simulink model "SingleWheelAug"  (R2025b)
settings: Solver=VariableStepAuto  StartTime=0.0  StopTime=10.0  RelTol=1e-3
undefined symbols (not defined in the file): InvDyn, ureal, uss
libraries: RCTblocks x2
settings Model: Creator=d.alazard  LastModifiedBy=andre
settings SolverCC: AlgebraicLoopSolver=TrustRegion
settings DebuggingCC: AlgebraicLoopMsg=none  UnconnectedInputMsg=warning  UnconnectedOutputMsg=warning  UnconnectedLineMsg=warning
settings ModelReferenceCC: EnableRefExpFcnMdlSchedulingChecks=on
settings RTWCC: GPUComputeCapability=3.5  DLArmComputeVersion=19.05

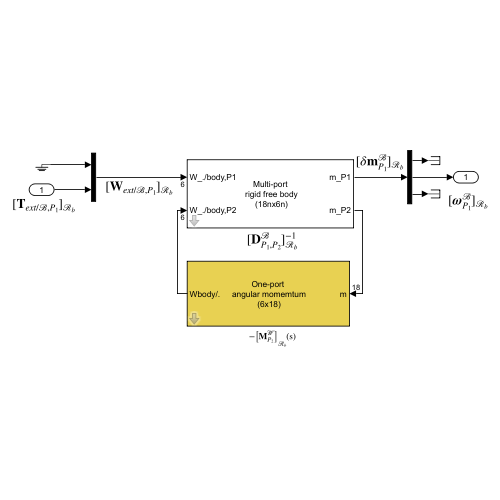
[thumbnail: Simulink's stored preview of the top-level diagram]
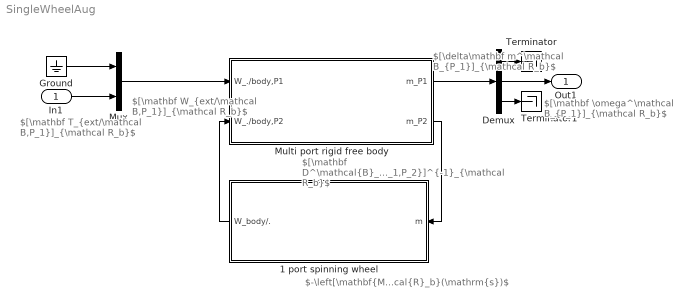
== system SingleWheelAug ==
  note: $-\left[\mathbf{M}^{\mathcal{W}}_{P_2}\right]_{\mathcal{R}_b}(\mathrm{s})$
  note: $[\mathbf W_{ext/\mathcal B,P_1}]_{\mathcal R_b}$
  note: $[\mathbf T_{ext/\mathcal B,P_1}]_{\mathcal R_b}$
  note: $[\delta\mathbf m^\mathcal B_{P_1}]_{\mathcal R_b}$
  note: $[\mathbf D^\mathcal{B}_{P_1,P_2}]^{-1}_{\mathcal R_b}$
  note: $[\mathbf \omega^\mathcal B_{P_1}]_{\mathcal R_b}$
  In1 : Inport
  1 port spinning wheel : Subsystem  mask(One-port spinning wheel (6x18)){ra=[0;0;1], m=0, Iw=0.1, Ir=0, OG=[0;0;0], OP=[0;0;0], Omega=100}
      mask prompts: ra "Wheel axis (3x1 vector)"; m "Wheel mass (Kg)"; Iw "Wheel axial Inertia  (at G, Kgm^2)"; Ir "Wheel radial inertia (at G, Kgm^2)"; OG "OG (3x1 vector, m)"; OP "OP (3x1 vector, m)"; Omega "spinning rate (rd/s)"
      mask help:
      | Dynamic model of an onboard angular momentum (spinning wheel) at point P (connection point with a parent body):
      | 6x18 transfer between motion vector  at P and wrench applied by this body at P.
      | 0: the reference point
      | G: the center of the wheel
      | P: the connection point
      |
      | All parameters are expressed in the (inherit) body frame.
      | Only the spinning rate can be an uncertain parameter declared with "ureal"
      mask init:
      | pass=ra2DCMi(ra);
      | Tau_GP=kinematic_model(OG,OP);
      mask Help: web('DocMomentum.html','-browser')
      mask DialogControl ParameterGroupVar Prompt: Main parameters
      mask Display:
      | disp('One-port\n angular momemtum\n (6x18)')
      | port_label('input', 1, 'm')
      | port_label('output', 1, 'Wbody/.')
  Demux : Demux  Outputs=[9 3 6]
  Ground : Ground
  Multi port rigid free body : Subsystem  mask(Multi-port rigid body (18nx6n)){m=1000, Ig=[75 1 2;1 40 -1;2 -1 80], OG=[0.35;1.5;0.5], n=2, OP1=[0;0;0], OP2=[0.35;1.5;0.5], OP3=[ureal('P3_y',1,'percent',10);0;0], OP4=[0;0;0], OP5=[0;0;0]}
      mask prompts: m "Mass (Kg)"; Ig "Inertia (at G, Kg m^2)"; OG "OG (3x1 vector, m)"; n "Number of ports"; OP1 "OP1 (3x1 vector, m)"; OP2 "OP2 (3x1 vector, m)"; OP3 "OP3 (3x1 vector, m)"; OP4 "OP4 (3x1 vector, m)"; OP5 "OP5 (3x1 vector,m)"
      mask help:
      | 18nx6n dynamic model of a rigid body at n given points (ports) between wrenches applied at the n points (input) and the motions vectors at these points (output).
      |
      | 0: the reference point
      | G: the center of mass
      | Pi (i=1:n): the n given connection points (n<6).
      |
      | All parameters are expressed in the body frame.
      | Each parameter can be an uncertain parameter declared with "ureal"
      mask init:
      | MultiPortRigidFreeBody
      mask Help: %web('Docmultiportrigidbody.html')
      mask TypeOptions n: 1 | 2 | 3 | 4 | 5
      mask DialogControl ParameterGroupVar Prompt: Main parameters
      mask DialogControl port1 Prompt: Port #1
      mask DialogControl port2 Prompt: #2
      mask DialogControl port3 Prompt: #3
      mask DialogControl port4 Prompt: #4
      mask DialogControl port5 Prompt: #5
      mask Display:
      | disp('Multi-port\n rigid free body\n (18nx6n)')
      | for ii=1:n
      |     port_label('input', ii,['W_./body,P',num2str(ii)])
      |     port_label('output',ii,['m_P',num2str(ii)])
      | end
  Mux : Mux  Inputs=[3 3]
  Terminator : Terminator
  Terminator1 : Terminator
  Out1 : Outport
  wires:
  1 port spinning wheel/1(W_body/.) -> Multi port rigid free body/2(W_./body,P2)
  Mux/1 -> Multi port rigid free body/1(W_./body,P1)
  Ground/1 -> Mux/1
  In1/1 -> Mux/2
  Multi port rigid free body/1(m_P1) -> Demux/1
  Demux/2 -> Out1/1
  Demux/1 -> Terminator/1
  Demux/3 -> Terminator1/1
  Multi port rigid free body/2(m_P2) -> 1 port spinning wheel/1(m)

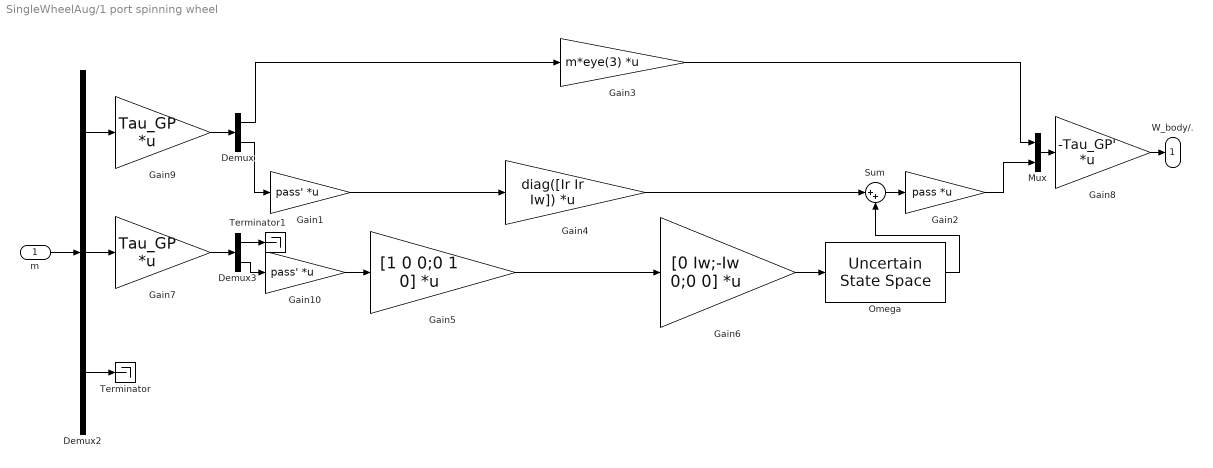
== system SingleWheelAug/1 port spinning wheel ==
  m : Inport  PortDimensions=18
  Demux : Demux  Outputs=[3 3]
  Demux2 : Demux  Outputs=[6 6 6]
  Demux3 : Demux  Outputs=[3 3]
  Gain1 : Gain  Gain=pass'  Multiplication=Matrix(K*u) (u vector)
  Gain10 : Gain  Gain=pass'  Multiplication=Matrix(K*u) (u vector)
  Gain2 : Gain  Gain=pass  Multiplication=Matrix(K*u) (u vector)
  Gain3 : Gain  Gain=m*eye(3)  Multiplication=Matrix(K*u) (u vector)
  Gain4 : Gain  Gain=diag([Ir Ir Iw])  Multiplication=Matrix(K*u) (u vector)
  Gain5 : Gain  Gain=[1 0 0;0 1 0]  Multiplication=Matrix(K*u) (u vector)
  Gain6 : Gain  Gain=[0 Iw;-Iw 0;0 0]  Multiplication=Matrix(K*u) (u vector)
  Gain7 : Gain  Gain=Tau_GP  Multiplication=Matrix(K*u) (u vector)
  Gain8 : Gain  Gain=-Tau_GP'  Multiplication=Matrix(K*u) (u vector)
  Gain9 : Gain  Gain=Tau_GP  Multiplication=Matrix(K*u) (u vector)
  Mux : Mux  Inputs=[3 3]
  Omega : RCTblocks/Uncertain State Space  Tag=USS  USystem=uss(Omega*eye(3))  UValue=[]  X0=[]  uX0=[]
  Sum : Sum  Inputs=|++
  Terminator : Terminator
  Terminator1 : Terminator
  W_body/. : Outport  VectorParamsAs1DForOutWhenUnconnected=off
  wires:
  Gain10/1 -> Gain5/1
  Demux3/2 -> Gain10/1
  Demux3/1 -> Terminator1/1
  Gain7/1 -> Demux3/1
  Demux2/3 -> Terminator/1
  Demux2/2 -> Gain7/1
  Demux2/1 -> Gain9/1
  m/1 -> Demux2/1
  Gain3/1 -> Mux/1
  Gain2/1 -> Mux/2
  Demux/1 -> Gain3/1
  Demux/2 -> Gain1/1
  Gain1/1 -> Gain4/1
  Gain4/1 -> Sum/1
  Sum/1 -> Gain2/1
  Gain5/1 -> Gain6/1
  Gain6/1 -> Omega/1
  Omega/1 -> Sum/2
  Gain8/1 -> W_body/./1
  Mux/1 -> Gain8/1
  Gain9/1 -> Demux/1

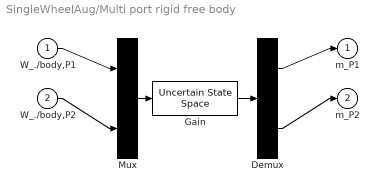
== system SingleWheelAug/Multi port rigid free body ==
  W_./body,P1 : Inport  PortDimensions=6
  W_./body,P2 : Inport  Port=2  PortDimensions=6
  Demux : Demux  Outputs=[18 18]
  Gain : RCTblocks/Uncertain State Space  Tag=USS  USystem=uss(InvDyn)  UValue=[]  X0=[]  uX0=[]
  Mux : Mux  Inputs=[6 6]
  m_P1 : Outport
  m_P2 : Outport  Port=2
  wires:
  Mux/1 -> Gain/1
  Gain/1 -> Demux/1
  W_./body,P1/1 -> Mux/1
  Demux/1 -> m_P1/1
  W_./body,P2/1 -> Mux/2
  Demux/2 -> m_P2/1
